simulink model "ee463q2"  (R2017a)
settings: Solver=FixedStepDiscrete  StartTime=0.0  StopTime=0.2  MaxStep=1e-4  RelTol=1e-3
libraries: powerlib x11, powerlib_meascontrol x3
settings Model: Creator=nailt  LastModifiedBy=nailt

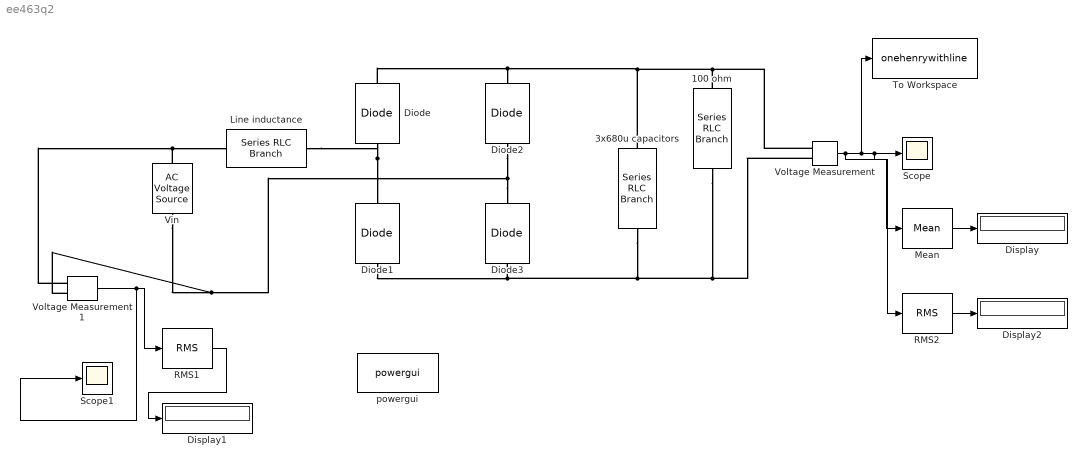
== system ee463q2 ==
  100 ohm : powerlib/Elements/Series RLC Branch  LConnTagsString=__new0  RConnTagsString=__new0  BranchType=RL  Resistance=25  Inductance=1e-3  SetiL0=off  InitialCurrent=0  Capacitance=1e-6  Setx0=off  InitialVoltage=0  Measurements=Branch voltage
  3x680u capacitors : powerlib/Elements/Series RLC Branch  LConnTagsString=__new0  RConnTagsString=__new0  BranchType=C  Resistance=1  Inductance=1e-3  SetiL0=off  InitialCurrent=0  Capacitance=2.04e-3  Setx0=off  InitialVoltage=0  Measurements=Branch voltage
  Diode : powerlib/Power Electronics/Diode  Ron=0.02  Lon=0  Vf=0.90  IC=0  UseSnubber=off  Rs=1e9  Cs=250e-9  Measurements=off
  Diode1 : powerlib/Power Electronics/Diode  Ron=0.02  Lon=0  Vf=0.90  IC=0  UseSnubber=off  Rs=1e9  Cs=250e-9  Measurements=off
  Diode2 : powerlib/Power Electronics/Diode  Ron=0.02  Lon=0  Vf=0.9  IC=0  UseSnubber=off  Rs=1e9  Cs=250e-9  Measurements=off
  Diode3 : powerlib/Power Electronics/Diode  Ron=0.02  Lon=0  Vf=0.90  IC=0  UseSnubber=off  Rs=1e9  Cs=250e-9  Measurements=off
  Display : Display
  Display1 : Display
  Display2 : Display
  Line inductance : powerlib/Elements/Series RLC Branch  LConnTagsString=__new0  RConnTagsString=__new0  BranchType=L  Inductance=1e-2  SetiL0=off  InitialCurrent=0  Setx0=off  InitialVoltage=0  Measurements=None
  Mean : powerlib_meascontrol/Measurements/Mean  Freq=50  Vinit=0  Ts=1e-6
  RMS1 : powerlib_meascontrol/Measurements/RMS  TrueRMS=on  Freq=50  RMSInit=0  Ts=1e-6
  RMS2 : powerlib_meascontrol/Measurements/RMS  TrueRMS=on  Freq=50  RMSInit=0  Ts=1e-6
  Scope : Scope
  Scope1 : Scope
  To Workspace : ToWorkspace  VariableName=onehenrywithline  SaveFormat=Timeseries  SampleTime=-1
  Vin : powerlib/Electrical Sources/AC Voltage Source  Amplitude=230*sqrt(2)  Phase=0  Frequency=50  SampleTime=0  Measurements=Voltage  BusType=swing  Pref=10e3  Qref=0  Qmin=-inf  Qmax=+inf
  Voltage Measurement : powerlib/Measurements/Voltage Measurement  PhasorSimulation=off  OutputType=Complex  PSBequivalent=0
  Voltage Measurement1 : powerlib/Measurements/Voltage Measurement  PhasorSimulation=off  OutputType=Complex  PSBequivalent=0
  powergui : powerlib/powergui  Priority=1  SimulationMode=Discrete  SampleTime=1e-6  frequency=60  Iterations=50  frequencyindice=50  Pbase=100e6  ErrMax=1e-4  UnitsV=kV  UnitsW=MW  buscounter=0  FunctionMessages=off  echomessages=off  EnableUseOfTLC=off  CurrentSourceSwitches=off  DisableSnubberDevices=off  DisableRonSwitches=off  DisableVfSwitches=off  DisplayEquations=off  SolverType=Tustin/Backward Euler (TBE)  Interpol=off  ExternalGateDelay=off  methode=off  Ts=100  x0status=blocks  SPID=on  SwTol=0  HookPort=off  RestoreLinks=warning  ResistiveCurrentMeasurement=off  Frange=[0:2:500]  Ylog=off  Xlog=on  ShowGrid=off  save=off  variable=ZData  structure=0  ZoomFFT=off  StartTime=0.0  cycles=1  DisplayStyle=1  fundamental=60  FreqAxis=off  MaxFrequency=1000  frequencyindicesteady=1  RmsSteady=1  display=off
  wires:
  RMS1/1 -> Display1/1
  Voltage Measurement/1 -> RMS2/1, To Workspace/1, Mean/1, Scope/1
  RMS2/1 -> Display2/1
  Mean/1 -> Display/1
  Voltage Measurement1/1 -> Scope1/1, RMS1/1
  connections:
  100 ohm/LConn1 -- Diode/RConn1 -- Diode2/RConn1 -- 3x680u capacitors/LConn1 -- Voltage Measurement/LConn1
  Vin/RConn1 -- Line inductance/LConn1 -- Voltage Measurement1/LConn1
  Diode3/RConn1 -- Diode2/LConn1 -- Voltage Measurement1/LConn2 -- Vin/LConn1
  100 ohm/RConn1 -- Diode1/LConn1 -- Diode3/LConn1 -- 3x680u capacitors/RConn1 -- Voltage Measurement/LConn2
  Line inductance/RConn1 -- Diode/LConn1 -- Diode1/RConn1
